simulink model "hw3_devs"  (R2014a)
settings: Solver=ode45  StartTime=0.0  StopTime=3000  RelTol=1e-3
undefined symbols (not defined in the file): des, gcbh
settings Model: Creator=feisele  LastModifiedBy=feisele

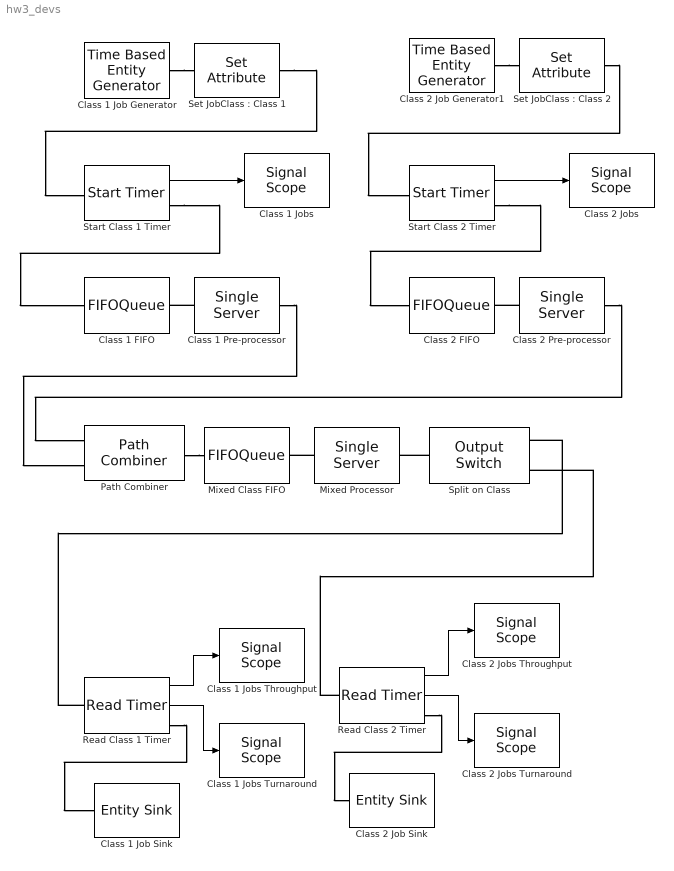
== system hw3_devs ==
  Class 1 Job Sink : EntitySink
  Class 1 Jobs Throughput : SignalScope  LoadFcn=des.scope.CallbackSupport('seLoadFcn',gcbh)  StartFcn=des.scope.CallbackSupport('seStartFcn',gcbh)  StopFcn=des.scope.CallbackSupport('seStopFcn',gcbh)  XMax=200  XLimitExceededOption=Keep axis limits unchanged  YLimitExceededOption=Keep axis limits unchanged  Title=Throughput for Class 1 Jobs  XLabel=time  YLabel=jobs processed
      settings: CopyFcn=des.scope.CallbackSupport('seCopyFcn',gcbh)  DeleteFcn=des.scope.CallbackSupport('seDeleteFcn',gcbh)  PreSaveFcn=des.scope.CallbackSupport('sePreSaveFcn',gcbh)  NameChangeFcn=des.scope.CallbackSupport('seNameChangeFcn',gcbh)  OpenFcn=des.scope.CallbackSupport('seOpenFcn',gcbh)  YMax=20
  "Class 1 Jobs Turnaround " : SignalScope  LoadFcn=des.scope.CallbackSupport('seLoadFcn',gcbh)  StartFcn=des.scope.CallbackSupport('seStartFcn',gcbh)  StopFcn=des.scope.CallbackSupport('seStopFcn',gcbh)  XMax=200  YLimitExceededOption=Keep axis limits unchanged  Title=Turnaround time for Class 1 Jobs  XLabel=time  YLabel=elapsed time (Class 1)
      settings: CopyFcn=des.scope.CallbackSupport('seCopyFcn',gcbh)  DeleteFcn=des.scope.CallbackSupport('seDeleteFcn',gcbh)  PreSaveFcn=des.scope.CallbackSupport('sePreSaveFcn',gcbh)  NameChangeFcn=des.scope.CallbackSupport('seNameChangeFcn',gcbh)  OpenFcn=des.scope.CallbackSupport('seOpenFcn',gcbh)  YMax=30
  Class 1 FIFO : FIFOQueue  Capacity=inf
  Class 1 Job Generator : TimeBasedEntityGenerator  Period=20  GenerateEntityAtSimulationStart=off  EntityType=Standard
  Class 1 Jobs : SignalScope  LoadFcn=des.scope.CallbackSupport('seLoadFcn',gcbh)  StartFcn=des.scope.CallbackSupport('seStartFcn',gcbh)  StopFcn=des.scope.CallbackSupport('seStopFcn',gcbh)  XMax=200  XLimitExceededOption=Keep axis limits unchanged  YLimitExceededOption=Keep axis limits unchanged  Title=Class 1 Job Submission  XLabel=time  YLabel=jobs submitted
      settings: CopyFcn=des.scope.CallbackSupport('seCopyFcn',gcbh)  DeleteFcn=des.scope.CallbackSupport('seDeleteFcn',gcbh)  PreSaveFcn=des.scope.CallbackSupport('sePreSaveFcn',gcbh)  NameChangeFcn=des.scope.CallbackSupport('seNameChangeFcn',gcbh)  OpenFcn=des.scope.CallbackSupport('seOpenFcn',gcbh)  YMax=20
  Class 1 Pre-processor : SingleServer  ServiceTime=5
  Class 2 Job Sink : EntitySink
  Class 2 Jobs Throughput : SignalScope  LoadFcn=des.scope.CallbackSupport('seLoadFcn',gcbh)  StartFcn=des.scope.CallbackSupport('seStartFcn',gcbh)  StopFcn=des.scope.CallbackSupport('seStopFcn',gcbh)  XMax=200  XLimitExceededOption=Keep axis limits unchanged  YLimitExceededOption=Keep axis limits unchanged  Title=Throughput for Class 2 Jobs  XLabel=time  YLabel=jobs processed
      settings: CopyFcn=des.scope.CallbackSupport('seCopyFcn',gcbh)  DeleteFcn=des.scope.CallbackSupport('seDeleteFcn',gcbh)  PreSaveFcn=des.scope.CallbackSupport('sePreSaveFcn',gcbh)  NameChangeFcn=des.scope.CallbackSupport('seNameChangeFcn',gcbh)  OpenFcn=des.scope.CallbackSupport('seOpenFcn',gcbh)  YMax=20
  Class 2 Jobs Turnaround : SignalScope  LoadFcn=des.scope.CallbackSupport('seLoadFcn',gcbh)  StartFcn=des.scope.CallbackSupport('seStartFcn',gcbh)  StopFcn=des.scope.CallbackSupport('seStopFcn',gcbh)  XMax=200  YLimitExceededOption=Keep axis limits unchanged  Title=Turnaround time for Class 2 Jobs  XLabel=time  YLabel=elapsed time (Class 2)
      settings: CopyFcn=des.scope.CallbackSupport('seCopyFcn',gcbh)  DeleteFcn=des.scope.CallbackSupport('seDeleteFcn',gcbh)  PreSaveFcn=des.scope.CallbackSupport('sePreSaveFcn',gcbh)  NameChangeFcn=des.scope.CallbackSupport('seNameChangeFcn',gcbh)  OpenFcn=des.scope.CallbackSupport('seOpenFcn',gcbh)  YMax=30
  Class 2 FIFO : FIFOQueue  Capacity=inf
  "Class 2 Job Generator1 " : TimeBasedEntityGenerator  Period=21  GenerateEntityAtSimulationStart=off  EntityType=Standard
  Class 2 Jobs : SignalScope  LoadFcn=des.scope.CallbackSupport('seLoadFcn',gcbh)  StartFcn=des.scope.CallbackSupport('seStartFcn',gcbh)  StopFcn=des.scope.CallbackSupport('seStopFcn',gcbh)  XMax=200  XLimitExceededOption=Keep axis limits unchanged  YLimitExceededOption=Keep axis limits unchanged  Title=Class 2 Job Submission  XLabel=time  YLabel=jobs submitted
      settings: CopyFcn=des.scope.CallbackSupport('seCopyFcn',gcbh)  DeleteFcn=des.scope.CallbackSupport('seDeleteFcn',gcbh)  PreSaveFcn=des.scope.CallbackSupport('sePreSaveFcn',gcbh)  NameChangeFcn=des.scope.CallbackSupport('seNameChangeFcn',gcbh)  OpenFcn=des.scope.CallbackSupport('seOpenFcn',gcbh)  YMax=20
  Class 2 Pre-processor : SingleServer  ServiceTime=7
  Mixed Class FIFO : FIFOQueue  Capacity=inf
  Mixed Processor : SingleServer  ServiceTime=10
  Path Combiner : PathCombiner  NumberInputPorts=2
  Read Class 1 Timer : ReadTimer  StatTimerNumberDeparted=on  StatTimeElapsed=on
      settings: OutputPortMap=o1,o2
  Read Class 2 Timer : ReadTimer  StatTimerNumberDeparted=on  StatTimeElapsed=on
      settings: OutputPortMap=o1,o2
  "Set JobClass : Class 1" : SetAttribute  AttributeName=JobClass  AttributeTreatAsVector=0  EvaluatedAttributeValue={ 1}
  "Set JobClass : Class 2" : SetAttribute  AttributeName=JobClass  AttributeValue=2  AttributeTreatAsVector=0  EvaluatedAttributeValue={ 2}
  Split on Class : OutputSwitch  NumberOutputPorts=2  SwitchingCriterion=From attribute  AttributeName=JobClass
  Start Class 1 Timer : StartTimer  StatNumberDeparted=on
  Start Class 2 Timer : StartTimer  StatNumberDeparted=on
  wires:
  Start Class 2 Timer/1 -> Class 2 Jobs/1
  Start Class 1 Timer/1 -> Class 1 Jobs/1
  Read Class 1 Timer/1 -> Class 1 Jobs Throughput/1
  Read Class 1 Timer/2 -> "Class 1 Jobs Turnaround "/1
  Read Class 2 Timer/1 -> Class 2 Jobs Throughput/1
  Read Class 2 Timer/2 -> Class 2 Jobs Turnaround/1
  connections:
  Class 1 Job Generator/RConn1 -- "Set JobClass : Class 1"/LConn1
  Start Class 1 Timer/RConn1 -- Class 1 FIFO/LConn1
  Class 1 Pre-processor/LConn1 -- Class 1 FIFO/RConn1
  Path Combiner/RConn1 -- Mixed Class FIFO/LConn1
  Class 1 Pre-processor/RConn1 -- Path Combiner/LConn2
  Class 2 Pre-processor/RConn1 -- Path Combiner/LConn1
  Class 2 Pre-processor/LConn1 -- Class 2 FIFO/RConn1
  Start Class 2 Timer/RConn1 -- Class 2 FIFO/LConn1
  "Set JobClass : Class 2"/RConn1 -- Start Class 2 Timer/LConn1
  Mixed Processor/LConn1 -- Mixed Class FIFO/RConn1
  Split on Class/LConn1 -- Mixed Processor/RConn1
  Read Class 1 Timer/RConn1 -- Class 1 Job Sink/LConn1
  Read Class 1 Timer/LConn1 -- Split on Class/RConn1
  Read Class 2 Timer/LConn1 -- Split on Class/RConn2
  Read Class 2 Timer/RConn1 -- Class 2 Job Sink/LConn1
  "Set JobClass : Class 1"/RConn1 -- Start Class 1 Timer/LConn1
  "Class 2 Job Generator1 "/RConn1 -- "Set JobClass : Class 2"/LConn1
